simulink model "pll"  (Simulink 6.0)
settings: Solver=ode45  StartTime=0.0  StopTime=0.15  RelTol=1e-3
libraries: commsynccomp2 x2, simulink x1
settings Model: LastModifiedBy=estel

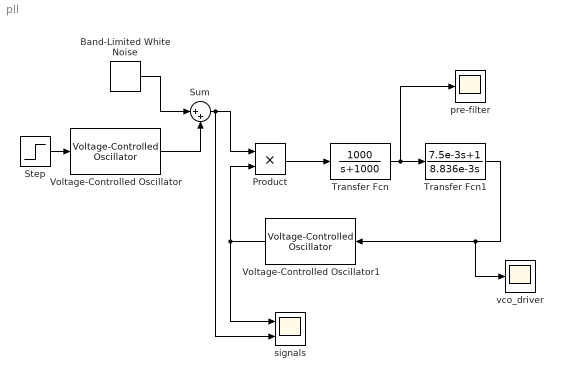
== system pll ==
  Band-Limited White Noise : simulink/Sources/Band-Limited White Noise  Cov=[0.00000]  Ts=3e-6  seed=[23341]
  Product : Product  RndMeth=Zero
  Step : Step  Time=10e-3  SampleTime=3e-6
  Sum : Sum  Inputs=|++
  Transfer Fcn : TransferFcn  Numerator=[1000]  Denominator=[1 1000]
  Transfer Fcn1 : TransferFcn  Numerator=[7.5e-3 1]  Denominator=[8.836e-3 0]
  Voltage-Controlled Oscillator : commsynccomp2/Voltage-Controlled Oscillator  Ac=1  Fc=5000  Kc=100  Ph=0
  Voltage-Controlled Oscillator1 : commsynccomp2/Voltage-Controlled Oscillator  Orientation=left  Ac=1  Fc=5000  Kc=70  Ph=0
  pre-filter : Scope
      settings: YMin=-1  YMax=2  SaveName=ScopeData2  SampleInput=on
  signals : Scope  NumInputPorts=2
      settings: TimeRange=0.000980392156865  YMin=-2~-2  YMax=2~2  SampleInput=on
  vco_driver : Scope
      settings: YMin=-1  YMax=2  SampleInput=on
  wires:
  Voltage-Controlled Oscillator1/1 -> Product/2, signals/1
  Product/1 -> Transfer Fcn/1
  Transfer Fcn/1 -> Transfer Fcn1/1, pre-filter/1
  Transfer Fcn1/1 -> Voltage-Controlled Oscillator1/1, vco_driver/1
  Step/1 -> Voltage-Controlled Oscillator/1
  Voltage-Controlled Oscillator/1 -> Sum/2
  Sum/1 -> Product/1, signals/2
  Band-Limited White Noise/1 -> Sum/1
